simulink model "optimasi_generic_algorithm"  (R2022a)
settings: Solver=VariableStepAuto  StartTime=0.0  StopTime=50  RelTol=1e-3
model workspace (MAT data in the model file):
  X = 1
undefined symbols (not defined in the file or in its folder): sigbuilder_block
settings Model: Creator=admin  LastModifiedBy=admin

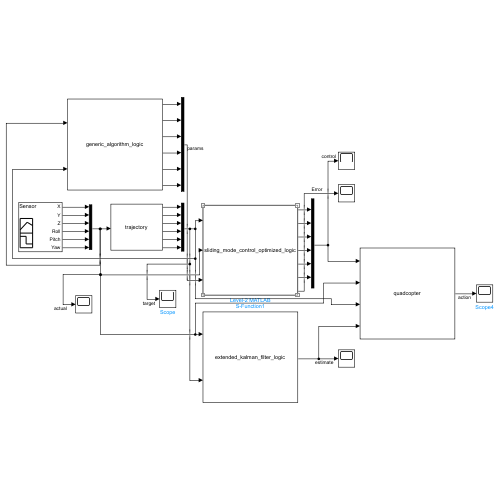
[thumbnail: Simulink's stored preview of the top-level diagram]
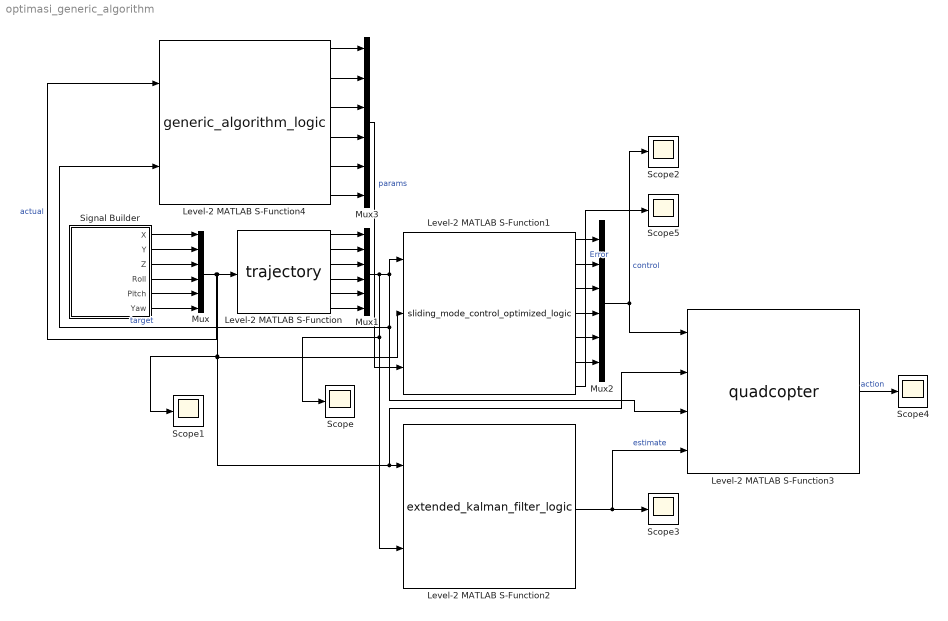
== system optimasi_generic_algorithm ==
  Level-2 MATLAB S-Function : M-S-Function  FunctionName=trajectory  Parameters=0,0,0,0
  Level-2 MATLAB S-Function1 : M-S-Function  FunctionName=sliding_mode_control_optimized_logic
  Level-2 MATLAB S-Function2 : M-S-Function  FunctionName=extended_kalman_filter_logic
  Level-2 MATLAB S-Function3 : M-S-Function  FunctionName=quadcopter
  Level-2 MATLAB S-Function4 : M-S-Function  FunctionName=generic_algorithm_logic
  Mux{,1..3} (4 alike) : Mux  Inputs=6
  Scope{,1..5} (6 alike) : Scope
  Signal Builder : Subsystem  Tag=STV Subsys  LoadFcn=sigbuilder_block('load');  StartFcn=sigbuilder_block('start');  StopFcn=sigbuilder_block('stop');  ClipboardFcn=sigbuilder_block('clipboard');  mask(Sigbuilder block){tuvar=[0:10]}
      mask help: Simulink:masks:SigbuilderBlock_MD
      mask init:
      | if ~strcmp(get_param(bdroot(gcbh),'SimulationStatus'),'stopped') tuvar = sigbuilder_block('maskInit'); end
      settings: CopyFcn=sigbuilder_block('copy');  DeleteFcn=sigbuilder_block('delete');  ModelCloseFcn=sigbuilder_block('modelClose');  PreSaveFcn=sigbuilder_block('preSave');  PauseFcn=sigbuilder_block('pause');  ContinueFcn=sigbuilder_block('continue');  NameChangeFcn=sigbuilder_block('namechange');  OpenFcn=sigbuilder_block('open',[337 58 543.5 463.5 ]);  CloseFcn=sigbuilder_block('close');
      mask Display: plot(0, 0, 100, 100,[2, 2, 32, 32, 2], [68, 8, 8, 68, 68],[32, 2], [38, 38], [32, 19, 2],[53, 60, 44], [32, 17, 17, 2],[16, 16, 31, 31]);txt = getActiveGroup(gcbh);text(2, 100, txt,'verticalAlignment', 'top');
  wires:
  Signal Builder/1(X) -> Mux/1
  Signal Builder/2(Y) -> Mux/2
  Signal Builder/3(Z) -> Mux/3
  Mux/1 -> Level-2 MATLAB S-Function4/1, Level-2 MATLAB S-Function3/2, Level-2 MATLAB S-Function2/1, Level-2 MATLAB S-Function1/2, Scope1/1, Level-2 MATLAB S-Function/1  "actual"
  Signal Builder/4(Roll) -> Mux/4
  Signal Builder/5(Pitch) -> Mux/5
  Signal Builder/6(Yaw) -> Mux/6
  Level-2 MATLAB S-Function/1 -> Mux1/1
  Level-2 MATLAB S-Function/2 -> Mux1/2
  Level-2 MATLAB S-Function/3 -> Mux1/3
  Level-2 MATLAB S-Function/4 -> Mux1/4
  Level-2 MATLAB S-Function/6 -> Mux1/6
  Level-2 MATLAB S-Function/5 -> Mux1/5
  Mux1/1 -> Level-2 MATLAB S-Function2/2, Scope/1, Level-2 MATLAB S-Function3/3, Level-2 MATLAB S-Function4/2, Level-2 MATLAB S-Function1/1  "target"
  Level-2 MATLAB S-Function1/1 -> Mux2/1
  Level-2 MATLAB S-Function1/2 -> Mux2/2
  Level-2 MATLAB S-Function1/3 -> Mux2/3
  Level-2 MATLAB S-Function1/4 -> Mux2/4
  Level-2 MATLAB S-Function1/5 -> Mux2/5
  Level-2 MATLAB S-Function1/6 -> Mux2/6
  Mux2/1 -> Level-2 MATLAB S-Function3/1, Scope2/1  "control"
  Level-2 MATLAB S-Function2/1 -> Level-2 MATLAB S-Function3/4, Scope3/1  "estimate"
  Level-2 MATLAB S-Function3/1 -> Scope4/1  "action"
  Level-2 MATLAB S-Function1/7 -> Scope5/1  "Error"
  Level-2 MATLAB S-Function4/1 -> Mux3/1
  Level-2 MATLAB S-Function4/2 -> Mux3/2
  Level-2 MATLAB S-Function4/3 -> Mux3/3
  Level-2 MATLAB S-Function4/4 -> Mux3/4
  Level-2 MATLAB S-Function4/5 -> Mux3/5
  Level-2 MATLAB S-Function4/6 -> Mux3/6
  Mux3/1 -> Level-2 MATLAB S-Function1/3  "params"

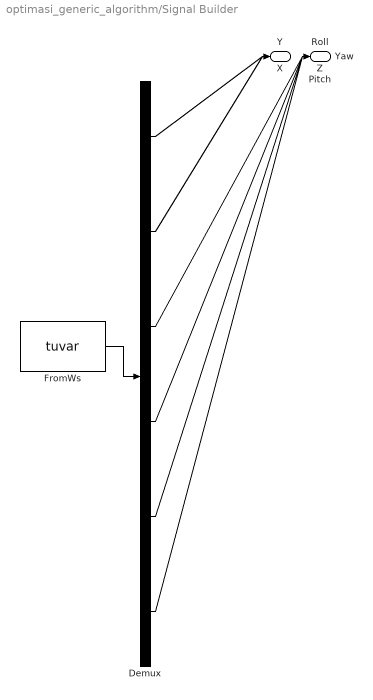
== system optimasi_generic_algorithm/Signal Builder ==
  Demux : Demux  Tag=STV Demux  Outputs=6
      settings: DisplayOption=none
  FromWs : FromWorkspace  Tag=STV FromWs  VariableName=tuvar
      SigBuilderData=|
      | common.afterFinalStr = 'Extrapolate'
      | common.sampleTime = 0
      | dataSet.timeRange = [0 30]
      | dataSet.name = 'Sensor'
      | sbobj.Groups.Name = 'Sensor'
      | sbobj.Groups.Signals(1).Name = 'X'
      | sbobj.Groups.Signals(1).XData = [0 1.54 1.54 2.96 6 30]
      | sbobj.Groups.Signals(1).YData = [0.005 0.005 0.4 0.405 1 1]
      | sbobj.Groups.Signals(2).Name = 'Y'
      | sbobj.Groups.Signals(2).XData = [0 2.86 4.82 6.56 10 30]
      | sbobj.Groups.Signals(2).YData = [-0.02 -0.75 -0.1 -0.62 -0.02 -0.02]
      | sbobj.Groups.Signals(3).Name = 'Z'
      | sbobj.Groups.Signals(3).XData = [0 1.02 2.9 4.62 10 30]
      | sbobj.Groups.Signals(3).YData = [0 0.2 0.3 0.2 0.3 0.3]
      | sbobj.Groups.Signals(4).Name = 'Roll'
      | sbobj.Groups.Signals(4).XData = [0 1.3 1.75 2.3 2.8 3.35 4.2 5 5 5.38 5.85 6.8 7.96 8.84 9.4 9.68 10 30]
      | sbobj.Groups.Signals(4).YData = [-0.03 0.09 0.05 0.17 0.05 0.07 0.07 -0.03 0.13 0.04 0.01 0.04 0.02 0.03 0.03 0.22 0.21 0.21]
      | sbobj.Groups.Signals(5).Name = 'Pitch'
      | sbobj.Groups.Signals(5).XData = [0 0.5 1.12 1.6 2.32 3.24 4.1 5 5 6.14 7.06 8.08 8.76 9.44 10 30]
      | sbobj.Groups.Signals(5).YData = [0 0.2 0.05 0.45 0.282926829268 0.15 0.5 0 0.5 0.4 0.2 0.05 0.7 0.45 1 1]
      | sbobj.Groups.Signals(6).Name = 'Yaw'
      | sbobj.Groups.Signals(6).XData = [0 5 5 30]
      | sbobj.Groups.Signals(6).YData = [0 0 1 1]
      | sbobj.Groups.TimeRange = [0 30]
  X : Outport  Tag=STV Outport
  Y : Outport  Tag=STV Outport  Port=2
  Z : Outport  Tag=STV Outport  Port=3
  Roll : Outport  Tag=STV Outport  Port=4
  Pitch : Outport  Tag=STV Outport  Port=5
  Yaw : Outport  Tag=STV Outport  Port=6
  wires:
  FromWs/1 -> Demux/1
  Demux/1 -> X/1
  Demux/2 -> Y/1
  Demux/3 -> Z/1
  Demux/4 -> Roll/1
  Demux/5 -> Pitch/1
  Demux/6 -> Yaw/1
